simulink model "Basic_Simulation"  (R2024b)
settings: Solver=FixedStepAuto  StartTime=0.0  StopTime=inf  RelTol=1e-3
undefined symbols (not defined in the file): Sim3dSensor
libraries: robotcorelib x2, eeGeneralControl x1, sim3dcameralib x1, sim3dlib x1, uavsim3dlib x1
settings Model: Creator=Sasha  LastModifiedBy=vince

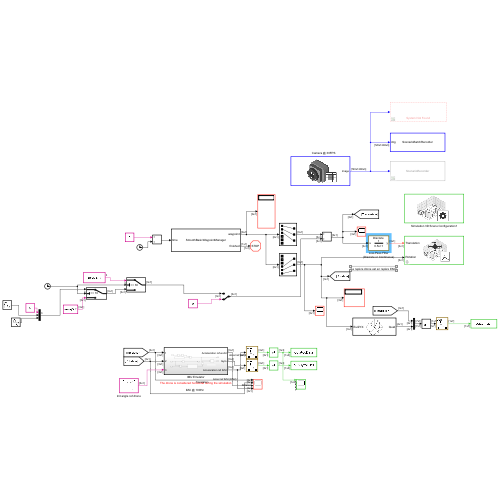
[thumbnail: Simulink's stored preview of the top-level diagram]
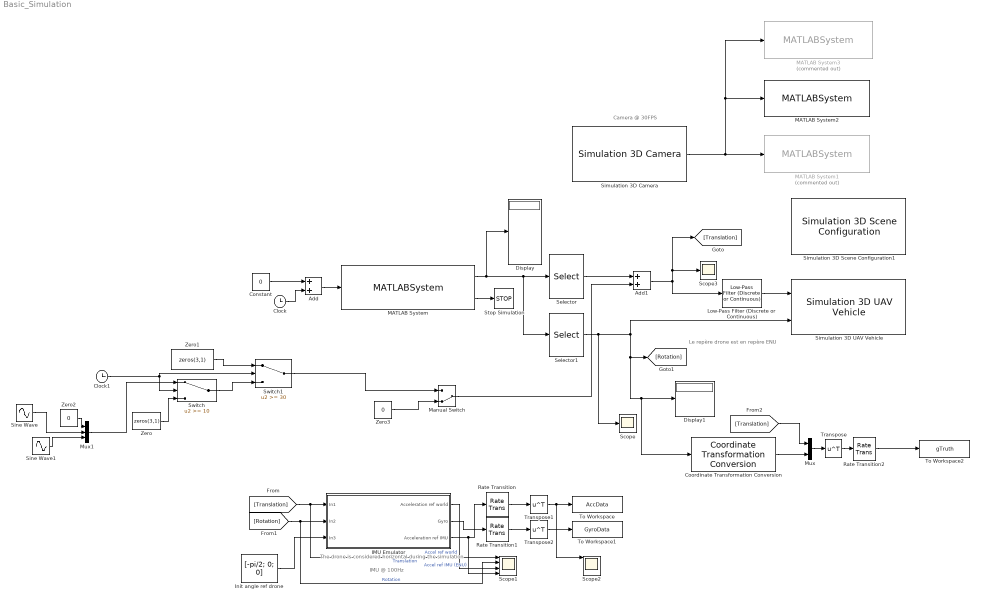
== system Basic_Simulation ==
  note: IMU @ 100Hz
  note: Camera @ 30FPS
  note: The drone is considered horizontal during the simulation
  note: Le repère drone est en repère ENU
  Add : Sum
  Add1 : Sum
  Clock : Clock
  Clock1 : Clock
  Constant : Constant  Value=0
  Coordinate Transformation Conversion : robotcorelib/Coordinate Transformation Conversion  InputRepresentation=Euler Angles  InputEulerSequence=ZYX  ShowTrVecInputPort=on  OutputRepresentation=Quaternion  OutputEulerSequence=ZYX  ShowTrVecOutputPort=on  SimulateUsing=Code generation
      settings: LibrarySourceBlock=navlib/Utilities/Coordinate Transformation Conversion
  Display : Display
  Display1 : Display
  IMU Emulator : Subsystem
  Init angle ref drone : Constant  Value=[-pi/2; 0; 0]  VectorParams1D=off
  Low-Pass Filter (Discrete or Continuous) : eeGeneralControl/Low-Pass Filter (Discrete or Continuous)  K=1  T=0.5  B=inf  A=-inf  init_option=Inherited from block input  x0=0  Ts=-1
  MATLAB System : MATLABSystem  System=SmoothBasicWaypointManager  ScenariosDirectory=C:\Users\vince\Documents\SEN5\CollaborativeSLAM\Scenarios  ScenarioName=8  StepTime=0.01  SimulateUsing=Interpreted execution
      mask Type: SmoothBasicWaypointManager
      mask Display:
      | disp('SmoothBasicWaypointManager');
      | port_label('input',1,'time');
      | port_label('output',1,'waypoint');
      | port_label('output',2,'finished');
  MATLAB System1 : MATLABSystem  Commented=on  System=ScenarioRecorder  ScenarioFrameDir=C:\Users\vince\Documents\SEN5\CollaborativeSLAM\Simulation\scenarios\4\images  SimulateUsing=Interpreted execution
      mask Type: ScenarioRecorder
      mask Display: disp('ScenarioRecorder');
  MATLAB System2 : MATLABSystem  System=ScenarioBatchRecorder  ScenariosDirectory=C:\Users\vince\Documents\SEN5\CollaborativeSLAM\Scenarios  ScenarioName=8  ImageSize=[ 720, 1280 ]  BufferSize=20  SimulateUsing=Interpreted execution
      mask Type: ScenarioBatchRecorder
      mask Display:
      | disp('ScenarioBatchRecorder');
      | port_label('input',1,'img');
  MATLAB System3 : MATLABSystem  Commented=on  System=AsyncScenarioBatchRecorder  ScenarioFrameDir=C:\Users\vince\Documents\SEN5\CollaborativeSLAM\v0\scenarios\4\images  ImageSize=[ 720, 1280 ]  BufferSize=10  SimulateUsing=Interpreted execution
  Manual Switch : ManualSwitch  CurrentSetting=0
  Mux : Mux  Inputs=2
  Mux1 : Mux  Inputs=3
  Rate Transition : RateTransition  OutPortSampleTime=0.01
  Rate Transition1 : RateTransition  OutPortSampleTime=0.01
  Rate Transition2 : RateTransition  OutPortSampleTime=0.01
  Scope : Scope
  Scope1 : Scope  NumInputPorts=4
  Scope2 : Scope  NumInputPorts=4
  Scope3 : Scope
  Selector : Selector  InputPortWidth=6  IndexOptions=Index vector (dialog)  Indices=[1 2 3]  OutputSizes=1
  Selector1 : Selector  InputPortWidth=6  IndexOptions=Index vector (dialog)  Indices=[4 5 6]  OutputSizes=1
  Simulation 3D Camera : sim3dcameralib/Simulation 3D Camera  Priority=1  sensorTag=Sim3dSensor�  sensorId=1  sensorName=Sim3dSensor�  vehTagList={'Scene Origin';'SimulinkVehicle1'}  vehTag=SimulinkVehicle1  mountLoc=Origin  offsetFlag=on  tmountOffset=[0, 0, 1]  extTmount=off  rmountOffset=[0, 0, 0]  extRmount=off  FocalLength=[1109, 1109]  OpticalCenter=[640, 360]  ImageSize=[720, 1280]  RadialDistortion=[0, 0]  TangentialDistortion=[0, 0]  SensorSkew=0  DepthOutportEnabled=off  SemanticOutportEnabled=off  TransformOutportEnabled=off  SampleTime=1/30  mountPoint=[0 0 1]  mountOrientation=[0 0 0]  aMode=3  ID=1
      settings: LibrarySourceBlock=drivingsim3d/Simulation 3D Camera
  Simulation 3D Scene Configuration1 : sim3dlib/Simulation 3D Scene Configuration  Priority=0  ProjectFormat=Default Scenes  SceneDesc=US city block  ProjectName=C:\Program Files\MATLAB\R2024b\toolbox\shared\sim3d_projects\automotive_project_windows\UE\WindowsNoEditor\VehicleSimulation.exe  ScenePath=/Game/Maps/USCityBlock  EnableOpenDRIVE=off  vehTagList={'Custom';'Scene Origin';'SimulinkVehicle1'}  vehTag=SimulinkVehicle1  FreeCameraInitialTranslation=[0, 0, 0]  FreeCameraDefaultInitialTranslation=[-6, 0, 2]  FreeCameraInitialRotation=[0, 0, 0]  FreeCameraDefaultInitialRotation=[0, -15, 0]  OpVisEn=off  Ts=1/100  EnableWindow=on  EnableRemoteAccess=off  EnableWeather=off  SunAzimuth=90  SunAltitude=40.0  EnableGeospatialSun=off  Latitude=0  Longitude=0  Date=2023-01-01  Time=10:30:00  GeoTimeZone=-5.0  SunDaylightSaving=off  wind=1  clouds=10  EnableVolumetricClouds=off  CloudCoverage=0  CloudAltitude=6  fog=0  rain=0  RaindropsEffect=off  SnowDensity=0  EnableGeospatial=off  UseTrueOrigin=off  OriginHeight=200  OriginLatitude=40.744652  OriginLongitude=-73.988864  MapStyle=Aerial  AdditionalAssetIDs=[]  UseAdvancedSunSky=off  SolarTime=11  TimeZone=-5  Day=21  Month=9  Year=2022  UseDaylightSavingTime=on  DSTStartDay=10  DSTStartMonth=3  DSTEndDay=3  DSTEndMonth=11  DSTSwitchHour=2  sensorTag=MainCamera2  sensorId=2  sensorName=MainCamera2  mountLoc=Origin  offsetFlag=off  tmountOffset=[0, 0, 0]  rmountOffset=[0, 0, 0]  HorizontalResolution=1280  VerticalResolution=720  HorizontalFOV=60  mountPoint=[0 0 0]  mountOrientation=[0 0 0]  aMode=4  ID=2  GeoTrigger=Inactive
      settings: LibrarySourceBlock=uavsim3dlib/Simulation 3D Scene Configuration
  Simulation 3D UAV Vehicle : uavsim3dlib/Simulation 3D UAV Vehicle  Priority=-1  Mesh=Quadrotor  MeshPath=/MathWorksUAVContent/UAVs/HexaRotorUAV/HexaRotor.HexaRotor  Color=Black  ActorName=SimulinkVehicle1  UseGlobalFrame=off  InitialTranslation=[0 0 0]  InitialRotation=[0 0 0]  InitialTranslationGlobal=[0 0 0]  InitialGeoOrigin=[0 0 0]  InitialRotationGlobal=[0 0 0]  SampleTime=1/100  ActorType=SimulinkVehicle  ID=1  aMode=4  ActorTag=SimulinkVehicle1
  Sine Wave : Sin  Frequency=2*pi/3  SampleTime=0
  Sine Wave1 : Sin  Frequency=2*pi/3  Phase=pi/2  SampleTime=0
  Stop Simulation : Stop
  Switch : Switch  Threshold=10  SaturateOnIntegerOverflow=off  InputSameDT=off
  Switch1 : Switch  Threshold=30  SaturateOnIntegerOverflow=off  InputSameDT=off
  To Workspace : ToWorkspace  VariableName=AccData  SaveFormat=Timeseries  SampleTime=-1
  To Workspace1 : ToWorkspace  VariableName=GyroData  SaveFormat=Timeseries  SampleTime=-1
  To Workspace2 : ToWorkspace  VariableName=gTruth  SaveFormat=Timeseries  SampleTime=-1
  Transpose : Math  Operator=transpose
  Transpose1 : Math  Operator=transpose
  Transpose2 : Math  Operator=transpose
  Zero : Constant  Value=zeros(3,1)  VectorParams1D=off  OutDataTypeStr=Inherit: Inherit via back propagation
  Zero1 : Constant  Value=zeros(3,1)  OutDataTypeStr=Inherit: Inherit via back propagation
  Zero2 : Constant  Value=0  OutDataTypeStr=Inherit: Inherit via back propagation
  Zero3 : Constant  Value=0  OutDataTypeStr=Inherit: Inherit via back propagation
  wires:
  Clock/1 -> Add/2
  MATLAB System/1 -> Selector1/1, Selector/1, Display/1
  Add/1 -> MATLAB System/1
  Constant/1 -> Add/1
  Selector1/1 -> Simulation 3D UAV Vehicle/2, [Rotation], Coordinate Transformation Conversion/1, Display1/1, Scope/1
  MATLAB System/2 -> Stop Simulation/1
  [Translation] -> Scope1/1, IMU Emulator/1(In1)  "Translation"
  [Rotation] -> Scope1/2, IMU Emulator/2(In2)  "Rotation"
  IMU Emulator/2(Gyro) -> Rate Transition1/1
  Rate Transition/1 -> Transpose1/1
  Rate Transition1/1 -> Transpose2/1
  Simulation 3D Camera/1 -> MATLAB System1/1, MATLAB System3/1, MATLAB System2/1
  Coordinate Transformation Conversion/1 -> Mux/2
  [Translation] -> Mux/1
  Mux/1 -> Transpose/1
  Rate Transition2/1 -> To Workspace2/1
  Transpose/1 -> Rate Transition2/1
  Transpose1/1 -> Scope2/1, To Workspace/1
  Transpose2/1 -> To Workspace1/1
  Init angle ref drone/1 -> IMU Emulator/3(In3)
  IMU Emulator/3(Acceleration ref IMU) -> Rate Transition/1, Scope1/4  "Accel ref IMU (ENU)"
  IMU Emulator/1(Acceleration ref world) -> Scope1/3  "Accel ref world"
  Switch/1 -> Switch1/3
  Zero1/1 -> Switch1/1
  Clock1/1 -> Switch/2, Switch1/2
  Sine Wave/1 -> Mux1/2
  Sine Wave1/1 -> Mux1/3
  Zero/1 -> Switch/3
  Mux1/1 -> Switch/1
  Selector/1 -> Add1/1
  Add1/1 -> Scope3/1, [Translation], Low-Pass Filter (Discrete or Continuous)/1
  Zero2/1 -> Mux1/1
  Switch1/1 -> Manual Switch/1
  Zero3/1 -> Manual Switch/2
  Manual Switch/1 -> Add1/2
  Low-Pass Filter (Discrete or Continuous)/1 -> Simulation 3D UAV Vehicle/1

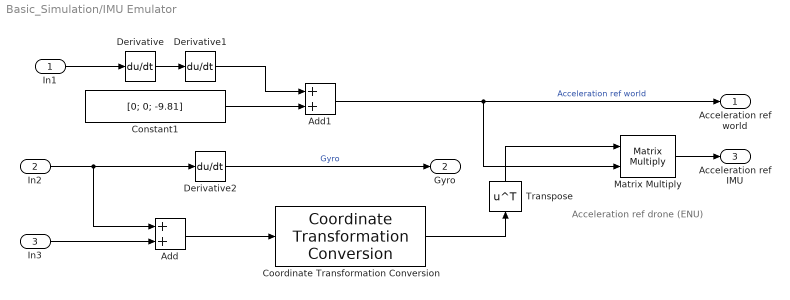
== system Basic_Simulation/IMU Emulator ==
  note: Acceleration ref drone (ENU)
  In1 : Inport
  In2 : Inport  Port=2
  In3 : Inport  Port=3
  Add : Sum
  Add1 : Sum
  Constant1 : Constant  Value=[0; 0; -9.81]
  Coordinate Transformation Conversion : robotcorelib/Coordinate Transformation Conversion  InputRepresentation=Euler Angles  InputEulerSequence=ZYX  ShowTrVecInputPort=on  OutputRepresentation=Rotation Matrix  OutputEulerSequence=ZYX  ShowTrVecOutputPort=on  SimulateUsing=Code generation
      settings: LibrarySourceBlock=navlib/Utilities/Coordinate Transformation Conversion
  Derivative : Derivative
  Derivative1 : Derivative
  Derivative2 : Derivative
  Matrix Multiply : Product  Multiplication=Matrix(*)
  Transpose : Math  Operator=transpose
  Acceleration ref world : Outport
  Gyro : Outport  Port=2
  Acceleration ref IMU : Outport  Port=3
  wires:
  Derivative/1 -> Derivative1/1
  Derivative2/1 -> Gyro/1  "Gyro"
  Constant1/1 -> Add1/2
  Add1/1 -> Matrix Multiply/2, Acceleration ref world/1  "Acceleration ref world"
  Derivative1/1 -> Add1/1
  In1/1 -> Derivative/1
  In2/1 -> Add/1, Derivative2/1
  In3/1 -> Add/2
  Add/1 -> Coordinate Transformation Conversion/1
  Matrix Multiply/1 -> Acceleration ref IMU/1
  Coordinate Transformation Conversion/1 -> Transpose/1
  Transpose/1 -> Matrix Multiply/1
